simulink model "pcc_dynamic_model_potential_force"  (R2021a)
settings: Solver=VariableStepAuto  StartTime=0.0  StopTime=30.0  MaxStep=0.005  RelTol=1e-3
libraries: simulink x3, simulink_extras x3
settings Model: Creator=maximilianstoelzle  LastModifiedBy=maximilianstoelzle

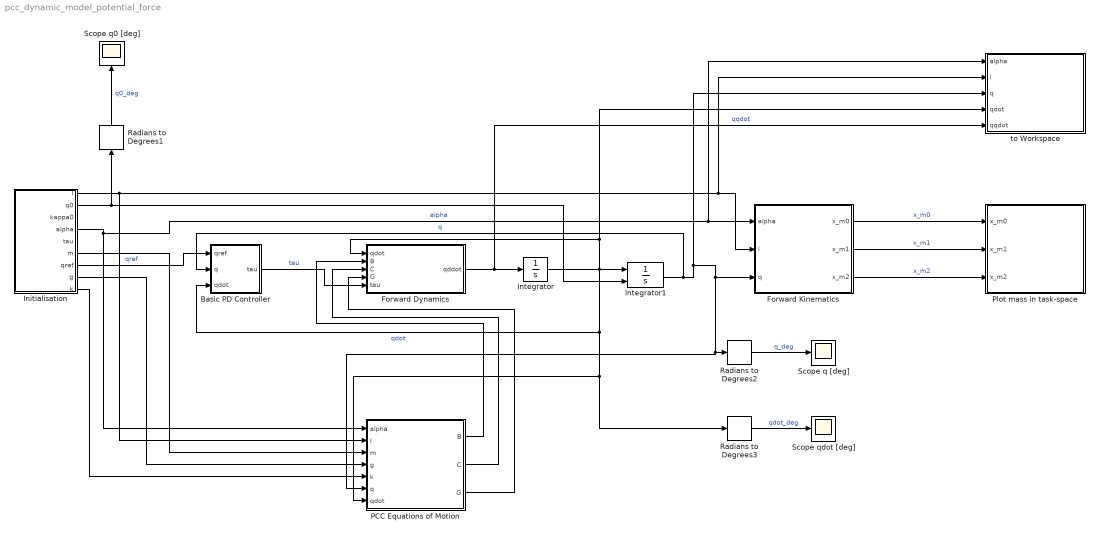
== system pcc_dynamic_model_potential_force ==
  Basic PD Controller : Subsystem
  Forward Dynamics : MATLAB Function  TreatAsAtomicUnit=on
  Forward Kinematics : MATLAB Function  TreatAsAtomicUnit=on
  Initialisation : Subsystem
  Integrator : Integrator  InitialCondition=[0; 0; 0]
  Integrator1 : Integrator  InitialConditionSource=external
  PCC Equations of Motion : MATLAB Function  TreatAsAtomicUnit=on
  Plot mass in task-space : Subsystem
  Radians to Degrees1 : simulink_extras/Transformations/Radians to Degrees
  Radians to Degrees2 : simulink_extras/Transformations/Radians to Degrees
  Radians to Degrees3 : simulink_extras/Transformations/Radians to Degrees
  Scope q [deg] : Scope
  Scope q0 [deg] : Scope
  Scope qdot [deg] : Scope
  to Workspace : Subsystem
  wires:
  Integrator/1 -> Forward Dynamics/1(qdot), to Workspace/4(qdot), Integrator1/1, Radians to Degrees3/1, PCC Equations of Motion/7(qdot), Basic PD Controller/3(qdot)  "qdot"
  Integrator1/1 -> Basic PD Controller/2(q), to Workspace/3(q), PCC Equations of Motion/6(q), Radians to Degrees2/1, Forward Kinematics/3(q)  "q"
  Radians to Degrees1/1 -> Scope q0 [deg]/1  "q0_deg"
  Radians to Degrees2/1 -> Scope q [deg]/1  "q_deg"
  PCC Equations of Motion/1(B) -> Forward Dynamics/2(B)
  PCC Equations of Motion/2(C) -> Forward Dynamics/3(C)
  PCC Equations of Motion/3(G) -> Forward Dynamics/4(G)
  Forward Dynamics/1(qddot) -> to Workspace/5(qqdot), Integrator/1  "qqdot"
  Forward Kinematics/1(x_m0) -> Plot mass in task-space/1(x_m0)  "x_m0"
  Forward Kinematics/2(x_m1) -> Plot mass in task-space/2(x_m1)  "x_m1"
  Forward Kinematics/3(x_m2) -> Plot mass in task-space/3(x_m2)  "x_m2"
  Initialisation/2(q0) -> Integrator1/2, Radians to Degrees1/1
  Initialisation/1(l) -> PCC Equations of Motion/2(l), Forward Kinematics/2(l), to Workspace/2(l)
  Initialisation/4(alpha) -> PCC Equations of Motion/1(alpha), to Workspace/1(alpha), Forward Kinematics/1(alpha)  "alpha"
  Initialisation/6(m) -> PCC Equations of Motion/3(m)
  Radians to Degrees3/1 -> Scope qdot [deg]/1  "qdot_deg"
  Initialisation/8(g) -> PCC Equations of Motion/4(g)
  Initialisation/7(qref) -> Basic PD Controller/1(qref)  "qref"
  Basic PD Controller/1(tau) -> Forward Dynamics/5(tau)  "tau"
  Initialisation/9(k) -> PCC Equations of Motion/5(k)

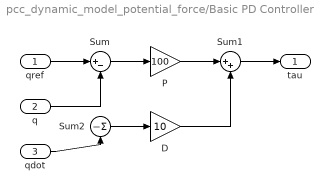
== system pcc_dynamic_model_potential_force/Basic PD Controller ==
  qref : Inport
  q : Inport  Port=2
  qdot : Inport  Port=3
  D : Gain  Gain=10
  P : Gain  Gain=100
  Sum : Sum  Inputs=|+-
  Sum1 : Sum  Inputs=|++
  Sum2 : Sum  Inputs=||-
  tau : Outport
  wires:
  qdot/1 -> Sum2/1
  Sum1/1 -> tau/1
  D/1 -> Sum1/2
  q/1 -> Sum/2
  qref/1 -> Sum/1
  Sum/1 -> P/1
  P/1 -> Sum1/1
  Sum2/1 -> D/1

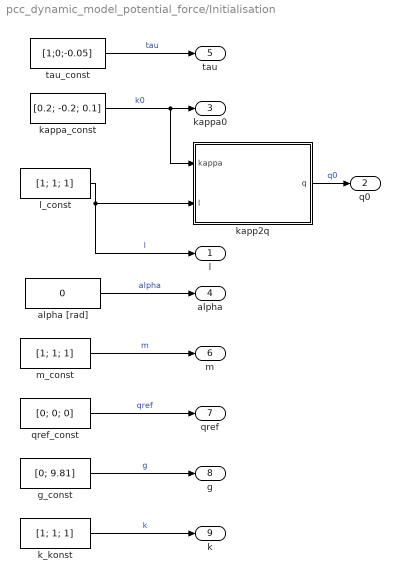
== system pcc_dynamic_model_potential_force/Initialisation ==
  alpha [rad] : Constant  Value=0
  g_const : Constant  Value=[0; 9.81]
  k_konst : Constant  Value=[1; 1; 1]
  kapp2q : MATLAB Function  TreatAsAtomicUnit=on
  kappa_const : Constant  Value=[0.2; -0.2; 0.1]
  l_const : Constant  Value=[1; 1; 1]
  m_const : Constant  Value=[1; 1; 1]
  qref_const : Constant  Value=[0; 0; 0]
  tau_const : Constant  Value=[1;0;-0.05]
  l : Outport
  q0 : Outport  Port=2
  kappa0 : Outport  Port=3
  alpha : Outport  Port=4
  tau : Outport  Port=5
  m : Outport  Port=6
  qref : Outport  Port=7
  g : Outport  Port=8
  k : Outport  Port=9
  wires:
  kappa_const/1 -> kapp2q/1(kappa), kappa0/1  "k0"
  l_const/1 -> kapp2q/2(l), l/1  "l"
  tau_const/1 -> tau/1  "tau"
  alpha [rad]/1 -> alpha/1  "alpha"
  kapp2q/1(q) -> q0/1  "q0"
  m_const/1 -> m/1  "m"
  qref_const/1 -> qref/1  "qref"
  g_const/1 -> g/1  "g"
  k_konst/1 -> k/1  "k"

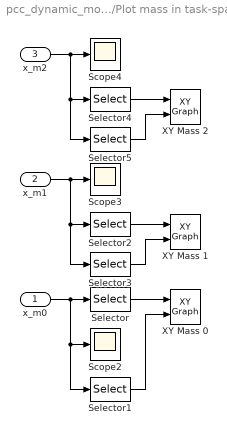
== system pcc_dynamic_model_potential_force/Plot mass in task-space ==
  x_m0 : Inport
  x_m1 : Inport  Port=2
  x_m2 : Inport  Port=3
  Scope2 : Scope
  Scope3 : Scope
  Scope4 : Scope
  Selector : Selector  InputPortWidth=2  IndexOptions=Index vector (dialog)  Indices=[1]  OutputSizes=1
  Selector1 : Selector  InputPortWidth=2  IndexOptions=Index vector (dialog)  Indices=[2]  OutputSizes=1
  Selector2 : Selector  InputPortWidth=2  IndexOptions=Index vector (dialog)  Indices=[1]  OutputSizes=1
  Selector3 : Selector  InputPortWidth=2  IndexOptions=Index vector (dialog)  Indices=[2]  OutputSizes=1
  Selector4 : Selector  InputPortWidth=2  IndexOptions=Index vector (dialog)  Indices=[1]  OutputSizes=1
  Selector5 : Selector  InputPortWidth=2  IndexOptions=Index vector (dialog)  Indices=[2]  OutputSizes=1
  XY Mass 0 : simulink/Sinks/XY Graph  xmin=-10  xmax=10  ymin=-10  ymax=10  st=-1
  XY Mass 1 : simulink/Sinks/XY Graph  xmin=-10  xmax=10  ymin=-10  ymax=10  st=-1
  XY Mass 2 : simulink/Sinks/XY Graph  xmin=-10  xmax=10  ymin=-10  ymax=10  st=-1
  wires:
  x_m2/1 -> Selector5/1, Selector4/1, Scope4/1
  Selector/1 -> XY Mass 0/1
  x_m1/1 -> Selector3/1, Selector2/1, Scope3/1
  Selector5/1 -> XY Mass 2/2
  Selector3/1 -> XY Mass 1/2
  Selector1/1 -> XY Mass 0/2
  x_m0/1 -> Scope2/1, Selector1/1, Selector/1
  Selector4/1 -> XY Mass 2/1
  Selector2/1 -> XY Mass 1/1

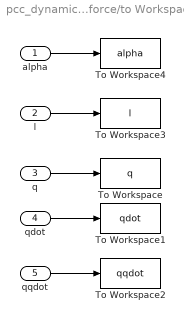
== system pcc_dynamic_model_potential_force/to Workspace ==
  alpha : Inport
  l : Inport  Port=2
  q : Inport  Port=3
  qdot : Inport  Port=4
  qqdot : Inport  Port=5
  To Workspace : ToWorkspace  VariableName=q  SaveFormat=Timeseries  SampleTime=-1
  To Workspace1 : ToWorkspace  VariableName=qdot  SaveFormat=Timeseries  SampleTime=-1
  To Workspace2 : ToWorkspace  VariableName=qqdot  SaveFormat=Timeseries  SampleTime=-1
  To Workspace3 : ToWorkspace  VariableName=l  SaveFormat=Timeseries  SampleTime=-1
  To Workspace4 : ToWorkspace  VariableName=alpha  SaveFormat=Timeseries  SampleTime=-1
  wires:
  alpha/1 -> To Workspace4/1
  qdot/1 -> To Workspace1/1
  l/1 -> To Workspace3/1
  qqdot/1 -> To Workspace2/1
  q/1 -> To Workspace/1

== matlab function pcc_dynamic_model_potential_force/Forward Kinematics ==
  data: alpha input; x_m0 output; l input; q input; x_m1 output; x_m2 output
function [x_m0, x_m1, x_m2] = forward_kinematics(alpha, l, q)
    x_m0 = q2xm0_fun(q, alpha, l);
    x_m1 = q2xm1_fun(q, alpha, l);
    x_m2 = q2xm2_fun(q, alpha, l);
end

== matlab function pcc_dynamic_model_potential_force/Forward Dynamics ==
  data: qdot input; B input; qddot output; C input; G input; tau input
function qddot  = forward_dynamics(qdot, B, C, G, tau)
    pinv_tol = 0.0001;
    qddot = pinv(B, pinv_tol)*(-C*qdot-G+tau);
end

== matlab function pcc_dynamic_model_potential_force/Initialisation/kapp2q ==
  data: kappa input; q output; l input
function q = kappa2q(kappa, l)
    q = [kappa(1) * l(1);
         kappa(2) * l(2);
         kappa(3) * l(3)];
end

== matlab function pcc_dynamic_model_potential_force/PCC Equations of Motion ==
  data: alpha input; l input; m input; B output; g input; k input; q input; qdot input; C output; G output
function [B, C, G]  = pcc_eom(alpha, l, m, g, k, q, qdot)
    B = B_fun(q, alpha, l, m);
    C = C_fun(q, qdot, alpha, l, m);
    G = G_fun(q, alpha, l, m, k, g);
end
